simulink model "Attitude_Control"  (R2021b)
settings: Solver=VariableStepAuto  StartTime=0.0  StopTime=Inf  FixedStep=0.001  RelTol=1e-3
values from neighbouring files (symbols this model uses):
  pitch_c = param(39)    [get_full_state.m]
  roll_c_1 = param(40)    [get_full_state.m]
  roll_c_2 = param(41)    [get_full_state.m]
undefined symbols (not defined in the file or in its folder): k_pitch, k_roll
libraries: vrlib x6, simulink_extras x3, matrix_library x3
settings Model: Creator=austm  LastModifiedBy=austm
settings SolverCC: ZeroCrossAlgorithm=Adaptive  AlgebraicLoopSolver=TrustRegion  AutoInsertRateTranBlk=on  InsertRTBMode=Never (minimum delay)  DecoupledContinuousIntegration=on  MinimalZcImpactIntegration=on
settings DataIOCC: ExternalInput=inputs0  InitialState=states  SaveFormat=Array  SaveOutput=off  SaveTime=off  ReturnWorkspaceOutputsName=tpc05cf441_1fa6_4e1e_817c_7c8b4b7bc3e9
settings OptimizationCC: EnhancedBackFolding=on  StrengthReduction=on  InitFltsAndDblsToZero=on  DifferentSizesBufferReuse=on
settings DebuggingCC: WriteAfterWriteMsg=DisableAll  AlgebraicLoopMsg=none  IgnoredZcDiagnostic=none  FcnCallInpInsideContextMsg=warning  UnconnectedInputMsg=none  UnconnectedOutputMsg=none  UnconnectedLineMsg=none  UniqueDataStoreMsg=error  RootOutportRequireBusObject=none  StateNameClashWarn=warning  StrictBusMsg=ErrorOnBusTreatedAsVector  SFUnexpectedBacktrackingDiag=warning  SFNoUnconditionalDefaultTransitionDiag=warning  SFExecutionAtInitializationDiag=none  SFMachineParentedDataDiag=warning  ArithmeticOperatorsInVariantConditions=warning
settings ModelReferenceCC: PropagateSignalLabelsOutOfModel=off
settings SFSimCC: SimUseLocalCustomCode=off
settings RTWCC: RTWUseLocalCustomCode=off
settings CodeAppCC: StateflowObjectComments=on

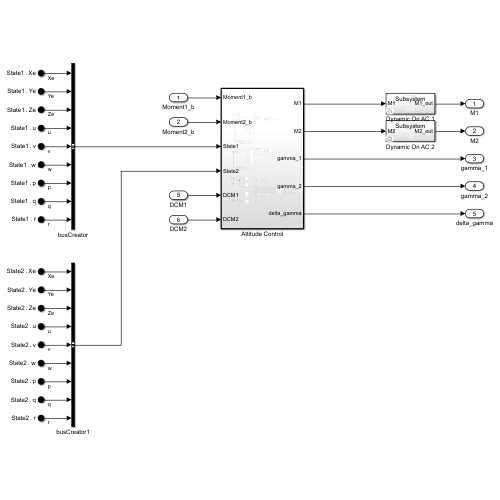
[thumbnail: Simulink's stored preview of the top-level diagram]
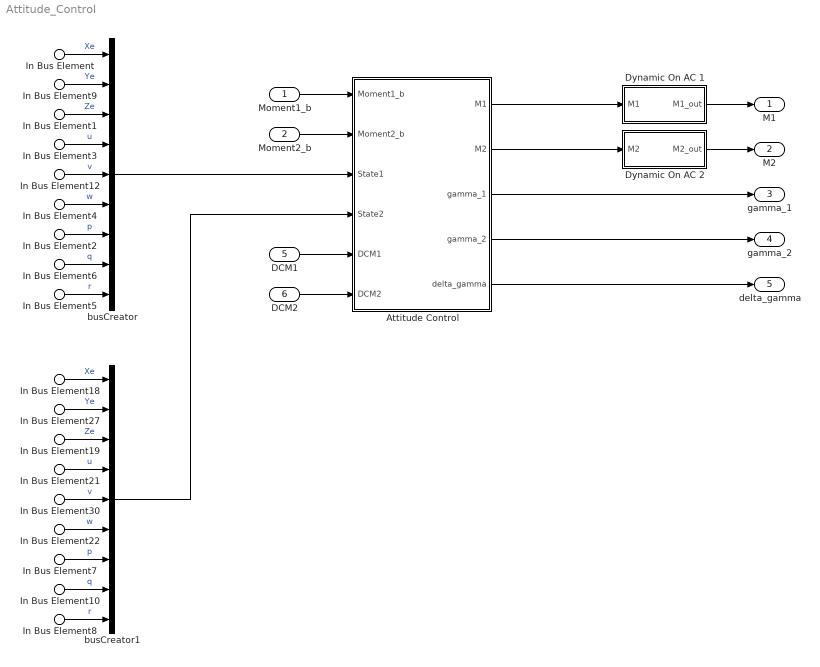
== system Attitude_Control ==
  Moment1_b : Inport  OutDataTypeStr=double  PortDimensions=3  SampleTime=0
  Moment2_b : Inport  Port=2  OutDataTypeStr=double  PortDimensions=3  SampleTime=0
  In Bus Element : Inport  Port=3  PortName=State1  Element=Xe
  In Bus Element1 : Inport  Port=3  PortName=State1  Element=Ze
  In Bus Element3 : Inport  Port=3  PortName=State1  Element=u
  In Bus Element4 : Inport  Port=3  PortName=State1  Element=w
  In Bus Element9 : Inport  Port=3  PortName=State1  Element=Ye
  In Bus Element12 : Inport  Port=3  PortName=State1  Element=v
  In Bus Element2 : Inport  Port=3  PortName=State1  Element=p
  In Bus Element6 : Inport  Port=3  PortName=State1  Element=q
  In Bus Element5 : Inport  Port=3  PortName=State1  Element=r
  In Bus Element18 : Inport  Port=4  PortName=State2  Element=Xe
  In Bus Element19 : Inport  Port=4  PortName=State2  Element=Ze
  In Bus Element21 : Inport  Port=4  PortName=State2  Element=u
  In Bus Element22 : Inport  Port=4  PortName=State2  Element=w
  In Bus Element27 : Inport  Port=4  PortName=State2  Element=Ye
  In Bus Element30 : Inport  Port=4  PortName=State2  Element=v
  In Bus Element7 : Inport  Port=4  PortName=State2  Element=p
  In Bus Element10 : Inport  Port=4  PortName=State2  Element=q
  In Bus Element8 : Inport  Port=4  PortName=State2  Element=r
  DCM1 : Inport  Port=5  OutDataTypeStr=double  PortDimensions=[3 3]  SampleTime=0
  DCM2 : Inport  Port=6  OutDataTypeStr=double  PortDimensions=[3 3]  SampleTime=0
  Attitude Control : Subsystem  TreatAsAtomicUnit=on
  Dynamic On AC 1 : Subsystem  Variant=on
  Dynamic On AC 2 : Subsystem  Variant=on
  busCreator : BusCreator  Inputs=9
  busCreator1 : BusCreator  Inputs=9
  M1 : Outport  OutDataTypeStr=double  PortDimensions=3  SampleTime=0
  M2 : Outport  Port=2  OutDataTypeStr=double  PortDimensions=3  SampleTime=0
  gamma_1 : Outport  Port=3  OutDataTypeStr=double  PortDimensions=3  SampleTime=0
  gamma_2 : Outport  Port=4  OutDataTypeStr=double  PortDimensions=3  SampleTime=0
  delta_gamma : Outport  Port=5  OutDataTypeStr=double  PortDimensions=3  SampleTime=0
  wires:
  DCM2/1 -> Attitude Control/6(DCM2)
  Moment1_b/1 -> Attitude Control/1(Moment1_b)
  Attitude Control/2(M2) -> Dynamic On AC 2/1(M2)
  DCM1/1 -> Attitude Control/5(DCM1)
  Attitude Control/1(M1) -> Dynamic On AC 1/1(M1)
  In Bus Element30/1 -> busCreator1/5  "v"
  In Bus Element27/1 -> busCreator1/2  "Ye"
  In Bus Element22/1 -> busCreator1/6  "w"
  In Bus Element21/1 -> busCreator1/4  "u"
  In Bus Element18/1 -> busCreator1/1  "Xe"
  In Bus Element19/1 -> busCreator1/3  "Ze"
  busCreator1/1 -> Attitude Control/4(State2)
  In Bus Element12/1 -> busCreator/5  "v"
  In Bus Element9/1 -> busCreator/2  "Ye"
  In Bus Element4/1 -> busCreator/6  "w"
  In Bus Element3/1 -> busCreator/4  "u"
  In Bus Element1/1 -> busCreator/3  "Ze"
  In Bus Element/1 -> busCreator/1  "Xe"
  busCreator/1 -> Attitude Control/3(State1)
  Moment2_b/1 -> Attitude Control/2(Moment2_b)
  Dynamic On AC 1/1(M1_out) -> M1/1
  Dynamic On AC 2/1(M2_out) -> M2/1
  In Bus Element2/1 -> busCreator/7  "p"
  In Bus Element6/1 -> busCreator/8  "q"
  In Bus Element5/1 -> busCreator/9  "r"
  In Bus Element7/1 -> busCreator1/7  "p"
  In Bus Element10/1 -> busCreator1/8  "q"
  In Bus Element8/1 -> busCreator1/9  "r"
  Attitude Control/3(gamma_1) -> gamma_1/1
  Attitude Control/4(gamma_2) -> gamma_2/1
  Attitude Control/5(delta_gamma) -> delta_gamma/1

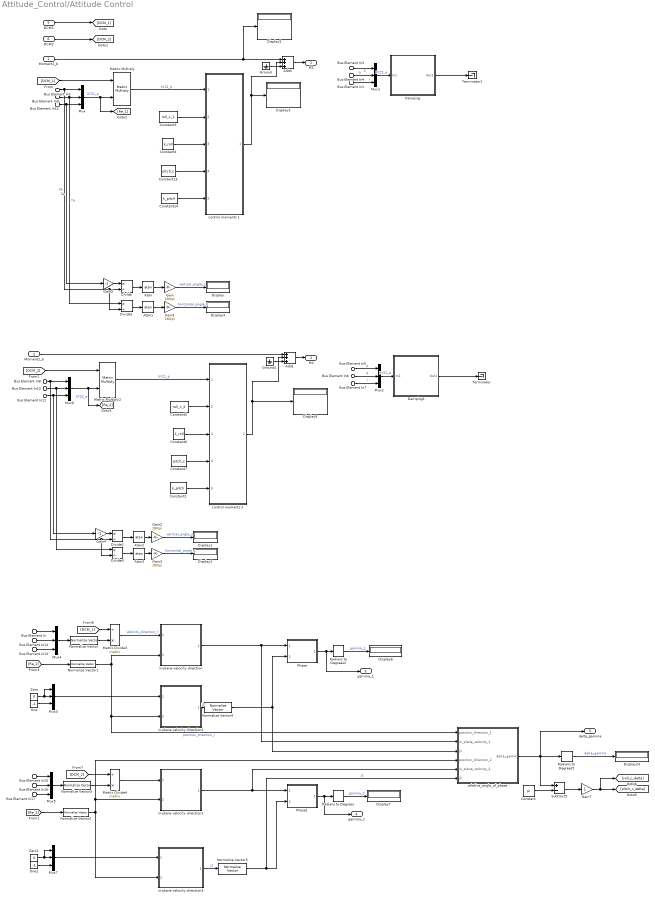
== system Attitude_Control/Attitude Control ==
  Moment1_b : Inport
  Moment2_b : Inport  Port=2
  Bus Element In12 : Inport  Port=3  PortName=State1  Element=Ze
  Bus Element In2 : Inport  Port=3  PortName=State1  Element=Xe
  Bus Element In9 : Inport  Port=3  PortName=State1  Element=Ye
  Bus Element In : Inport  Port=3  PortName=State1  Element=u
  Bus Element In13 : Inport  Port=3  PortName=State1  Element=w
  Bus Element In14 : Inport  Port=3  PortName=State1  Element=v
  Bus Element In3 : Inport  Port=3  PortName=State1  Element=p
  Bus Element In4 : Inport  Port=3  PortName=State1  Element=q
  Bus Element In1 : Inport  Port=3  PortName=State1  Element=r
  Bus Element In8 : Inport  Port=4  PortName=State2  Element=Xe
  Bus Element In10 : Inport  Port=4  PortName=State2  Element=Ye
  Bus Element In11 : Inport  Port=4  PortName=State2  Element=Ze
  Bus Element In15 : Inport  Port=4  PortName=State2  Element=u
  Bus Element In16 : Inport  Port=4  PortName=State2  Element=v
  Bus Element In17 : Inport  Port=4  PortName=State2  Element=w
  Bus Element In5 : Inport  Port=4  PortName=State2  Element=p
  Bus Element In6 : Inport  Port=4  PortName=State2  Element=q
  Bus Element In7 : Inport  Port=4  PortName=State2  Element=r
  DCM1 : Inport  Port=5
  DCM2 : Inport  Port=6
  Add1 : Sum  Inputs=+++
  Add3 : Sum  Inputs=+++
  Atan{,1..3} (4 alike) : Trigonometry  Operator=atan
  Constant : Constant  Value=pi
  Constant13 : Constant  Value=pitch_c
  Constant14 : Constant  Value=k_pitch
  Constant2 : Constant  Value=k_pitch
  Constant3 : Constant  Value=roll_c_1
  Constant4 : Constant  Value=k_roll
  Constant5 : Constant  Value=roll_c_2
  Constant6 : Constant  Value=k_roll
  Constant7 : Constant  Value=pitch_c
  Damping : Subsystem
  Damping1 : Subsystem
  Display{,1..8,24} (10 alike) : Display
  Divide{,1..3} (4 alike) : Product  Inputs=*/
  Gain{,1..3} (4 alike) : Gain  Gain=180/pi
  Gain4 : Gain  Gain=-1
  Gain5 : Gain  Gain=-1
  Gain7 : Gain
  Ground : Ground
  Ground1 : Ground
  Matrix Divide3 : Product  Inputs=/*  Multiplication=Matrix(*)
  Matrix Divide4 : Product  Inputs=/*  Multiplication=Matrix(*)
  Matrix Multiply : Product  Multiplication=Matrix(*)
  Matrix Multiply2 : Product  Multiplication=Matrix(*)
  Mux{,1..7} (8 alike) : Mux  Inputs=3
  Normalize Vector{,1..5} (6 alike) : vrlib/Utilities/Normalize Vector  maxzero=0
  One : Constant  Value=-1  OutDataTypeStr=Inherit: Inherit via back propagation
  One1 : Constant  Value=-1  OutDataTypeStr=Inherit: Inherit via back propagation
  Phase : Subsystem  ReferencedSubsystem=Phase
  Phase1 : Subsystem  ReferencedSubsystem=Phase
  Radians to Degrees : simulink_extras/Transformations/Radians to Degrees
  Radians to Degrees2 : simulink_extras/Transformations/Radians to Degrees
  Radians to Degrees5 : simulink_extras/Transformations/Radians to Degrees
  Subtract5 : Sum  Inputs=+-
  Terminator : Terminator
  Terminator1 : Terminator
  Zero : Constant  Value=0  OutDataTypeStr=Inherit: Inherit via back propagation
  Zero1 : Constant  Value=0  OutDataTypeStr=Inherit: Inherit via back propagation
  control moments 1 : Subsystem  ReferencedSubsystem=control_moments
  control moments 2 : Subsystem  ReferencedSubsystem=control_moments
  in-plane velocity direction{,1..3} (4 alike) : Subsystem  ReferencedSubsystem=in_plane_velocity_direction
  relative_angle_of_phase : Subsystem
  M1 : Outport
  M2 : Outport  Port=2
  gamma_1 : Outport  Port=3
  gamma_2 : Outport  Port=4
  delta_gamma : Outport  Port=5
  wires:
  relative_angle_of_phase/1(delta_gamma) -> delta_gamma/1, Subtract5/1, Radians to Degrees5/1
  Phase/1 -> gamma_1/1, Radians to Degrees2/1
  Mux7/1 -> in-plane velocity direction3/1
  Matrix Divide4/1 -> in-plane velocity direction1/1
  Mux3/1 -> in-plane velocity direction2/1
  in-plane velocity direction2/1 -> Normalize Vector4/1  "j1"
  Matrix Divide3/1 -> in-plane velocity direction/1  "velocity_direction_I"
  in-plane velocity direction/1 -> relative_angle_of_phase/2(in_plane_velocity_1), Phase/1
  Gain7/1 -> [pitch_c_delta], [roll_c_delta]
  Subtract5/1 -> Gain7/1
  Constant7/1 -> control moments 2/4
  Constant/1 -> Subtract5/2
  Radians to Degrees5/1 -> Display24/1  "delta_gamma"
  Normalize Vector1/1 -> in-plane velocity direction/2, in-plane velocity direction2/2, relative_angle_of_phase/1(position_direction_1)  "position_direction_I"
  Phase1/1 -> gamma_2/1, Radians to Degrees/1
  in-plane velocity direction1/1 -> relative_angle_of_phase/5(in_plane_velocity_2), Phase1/1
  Radians to Degrees/1 -> Display7/1  "gamma_2"
  Radians to Degrees2/1 -> Display6/1  "gamma_1"
  Normalize Vector5/1 -> Phase1/2, relative_angle_of_phase/6(j2)  "j2"
  Normalize Vector2/1 -> relative_angle_of_phase/4(position_direction_2), in-plane velocity direction1/2, in-plane velocity direction3/2
  One1/1 -> Mux7/3
  Zero1/1 -> Mux7/2, Mux7/1
  Zero/1 -> Mux3/2, Mux3/1
  One/1 -> Mux3/3
  Normalize Vector3/1 -> Matrix Divide4/2
  [Re_2] -> Normalize Vector2/1
  [Re_1] -> Normalize Vector1/1
  Normalize Vector/1 -> Matrix Divide3/2
  [DCM_1] -> Matrix Divide3/1
  Bus Element In14/1 -> Mux4/2
  [DCM_2] -> Matrix Divide4/1
  Mux5/1 -> Normalize Vector3/1
  Bus Element In17/1 -> Mux5/3
  Mux4/1 -> Normalize Vector/1
  Bus Element In/1 -> Mux4/1
  Bus Element In15/1 -> Mux5/1
  Bus Element In16/1 -> Mux5/2
  Bus Element In13/1 -> Mux4/3
  Atan/1 -> Gain/1
  Gain5/1 -> Divide/1
  Gain4/1 -> Divide2/1
  Gain2/1 -> Display1/1  "vertical_angle_2"
  Atan2/1 -> Gain2/1
  Atan3/1 -> Gain3/1
  Gain3/1 -> Display2/1  "horizontal_angle_2"
  Gain1/1 -> Display4/1  "horizontal_angle_1"
  Atan1/1 -> Gain1/1
  Gain/1 -> Display/1  "vertical_angle_1"
  Divide3/1 -> Atan3/1
  Divide2/1 -> Atan2/1
  Divide1/1 -> Atan1/1
  Divide/1 -> Atan/1
  Constant2/1 -> control moments 2/5
  Constant6/1 -> control moments 2/3
  Constant5/1 -> control moments 2/2
  Constant14/1 -> control moments 1/5
  Constant13/1 -> control moments 1/4
  Constant4/1 -> control moments 1/3
  Constant3/1 -> control moments 1/2
  control moments 2/1 -> Add1/2, Display8/1
  Matrix Multiply2/1 -> control moments 2/1  "XYZ1_b"
  Add3/1 -> M1/1
  control moments 1/1 -> Display3/1, Add3/2
  Matrix Multiply/1 -> control moments 1/1  "XYZ1_b"
  [DCM_2] -> Matrix Multiply2/1
  Bus Element In11/1 -> Mux6/3, Gain4/1
  Bus Element In10/1 -> Mux6/2, Divide3/1
  Bus Element In8/1 -> Mux6/1, Divide3/2, Divide2/2
  Add1/1 -> M2/1
  Mux6/1 -> Matrix Multiply2/2, [Re_2]  "XYZ2_e"
  Moment1_b/1 -> Add3/1, Display5/1
  DCM2/1 -> [DCM_2]
  DCM1/1 -> [DCM_1]
  Bus Element In2/1 -> Mux/1, Divide/2, Divide1/2  "Xe"
  Bus Element In12/1 -> Mux/3, Gain5/1  "Ze"
  Bus Element In9/1 -> Mux/2, Divide1/1  "Ye"
  Mux/1 -> Matrix Multiply/2, [Re_1]  "XYZ1_e"
  [DCM_1] -> Matrix Multiply/1
  Moment2_b/1 -> Add1/1
  Normalize Vector4/1 -> Phase/2, relative_angle_of_phase/3(j1)
  in-plane velocity direction3/1 -> Normalize Vector5/1  "j2"
  Bus Element In3/1 -> Mux1/1  "p"
  Bus Element In4/1 -> Mux1/2  "q"
  Bus Element In1/1 -> Mux1/3  "r"
  Mux1/1 -> Damping/1(In1)  "XYZ1_e"
  Damping/1(Out1) -> Terminator1/1
  Mux2/1 -> Damping1/1(In1)  "XYZ1_e"
  Bus Element In6/1 -> Mux2/2  "q"
  Bus Element In7/1 -> Mux2/3  "r"
  Bus Element In5/1 -> Mux2/1  "p"
  Damping1/1(Out1) -> Terminator/1
  Ground/1 -> Add3/3
  Ground1/1 -> Add1/3

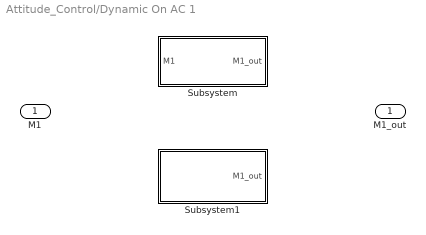
== system Attitude_Control/Dynamic On AC 1 ==
  M1 : Inport
  Subsystem : Subsystem  VariantControl=ac1_moments > 0
  Subsystem1 : Subsystem  VariantControl="ac1_moments ==  0"
  M1_out : Outport

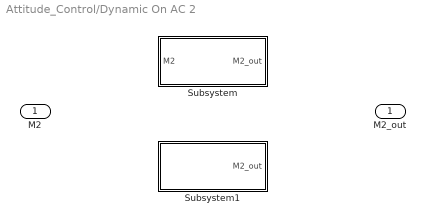
== system Attitude_Control/Dynamic On AC 2 ==
  M2 : Inport
  Subsystem : Subsystem  VariantControl=ac2_moments > 0
  Subsystem1 : Subsystem  VariantControl=ac2_moments == 0
  M2_out : Outport

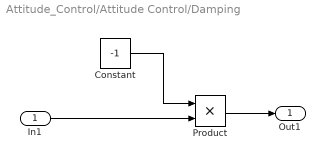
== system Attitude_Control/Attitude Control/Damping ==
  In1 : Inport
  Constant : Constant  Value=-1
  Product : Product
  Out1 : Outport
  wires:
  In1/1 -> Product/2
  Product/1 -> Out1/1
  Constant/1 -> Product/1

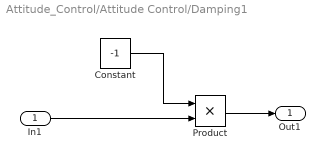
== system Attitude_Control/Attitude Control/Damping1 ==
  In1 : Inport
  Constant : Constant  Value=-1
  Product : Product
  Out1 : Outport
  wires:
  In1/1 -> Product/2
  Product/1 -> Out1/1
  Constant/1 -> Product/1

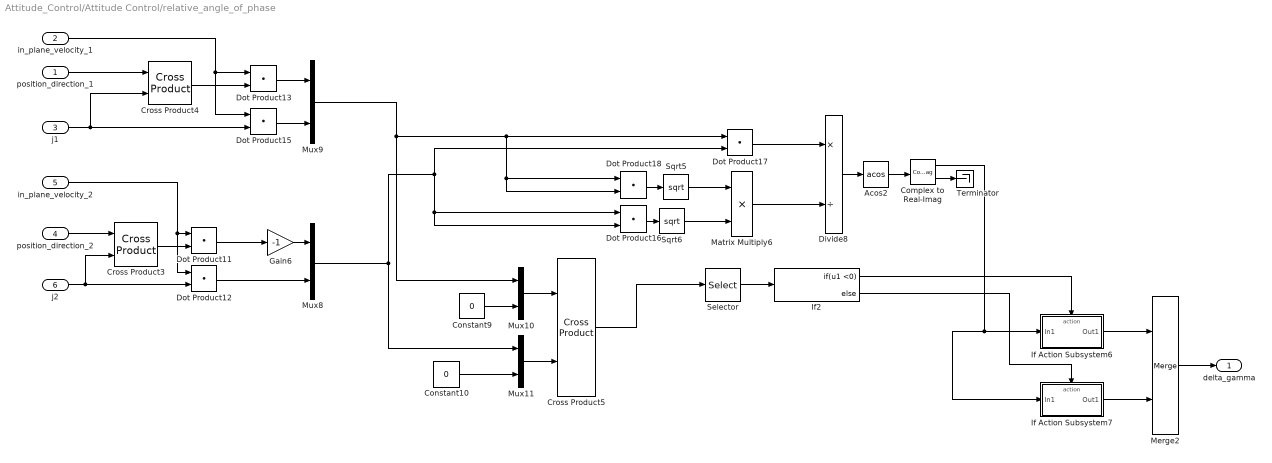
== system Attitude_Control/Attitude Control/relative_angle_of_phase ==
  position_direction_1 : Inport
  in_plane_velocity_1 : Inport  Port=2
  j1 : Inport  Port=3
  position_direction_2 : Inport  Port=4
  in_plane_velocity_2 : Inport  Port=5
  j2 : Inport  Port=6
  Acos2 : Trigonometry  Operator=acos  OutputSignalType=complex
  Complex to Real-Imag : ComplexToRealImag
  Constant10 : Constant  Value=0
  Constant9 : Constant  Value=0
  Cross Product3 : matrix_library/Cross Product
      settings: SourceProductBaseCode=SL
  Cross Product4 : matrix_library/Cross Product
      settings: SourceProductBaseCode=SL
  Cross Product5 : matrix_library/Cross Product
      settings: SourceProductBaseCode=SL
  Divide8 : Product  Inputs=*/
  Dot Product{11..13,15..18} (7 alike) : DotProduct  InputSameDT=on  OutDataTypeStr=Inherit: Inherit via internal rule
  Gain6 : Gain  Gain=-1
  If Action Subsystem6 : Subsystem  TreatAsAtomicUnit=on
  If Action Subsystem7 : Subsystem  TreatAsAtomicUnit=on
  If2 : If  IfExpression=u1 <0
  Matrix Multiply6 : Product
  Merge2 : Merge
  Mux{8..11} (4 alike) : Mux  Inputs=2
  Selector : Selector  InputPortWidth=3  IndexOptions=Index vector (dialog)  Indices=3  OutputSizes=1
  Sqrt5 : Sqrt  SaturateOnIntegerOverflow=on
  Sqrt6 : Sqrt  SaturateOnIntegerOverflow=on
  Terminator : Terminator
  delta_gamma : Outport
  wires:
  Acos2/1 -> Complex to Real-Imag/1
  Complex to Real-Imag/2 -> Terminator/1
  j1/1 -> Dot Product15/2, Cross Product4/2
  If Action Subsystem7/1(Out1) -> Merge2/2
  Dot Product15/1 -> Mux9/2
  If Action Subsystem6/1(Out1) -> Merge2/1
  Mux10/1 -> Cross Product5/1
  Constant9/1 -> Mux10/2
  Dot Product17/1 -> Divide8/1
  Cross Product5/1 -> Selector/1
  j2/1 -> Dot Product12/2, Cross Product3/2
  Mux11/1 -> Cross Product5/2
  Dot Product16/1 -> Sqrt6/1
  Merge2/1 -> delta_gamma/1
  in_plane_velocity_1/1 -> Dot Product15/1, Dot Product13/1
  If2/1 -> If Action Subsystem6/Action
  Sqrt6/1 -> Matrix Multiply6/2
  position_direction_2/1 -> Cross Product3/1
  Sqrt5/1 -> Matrix Multiply6/1
  Complex to Real-Imag/1 -> If Action Subsystem6/1(In1), If Action Subsystem7/1(In1)
  position_direction_1/1 -> Cross Product4/1
  Matrix Multiply6/1 -> Divide8/2
  Cross Product4/1 -> Dot Product13/2
  Divide8/1 -> Acos2/1
  Gain6/1 -> Mux8/1
  Selector/1 -> If2/1
  Dot Product18/1 -> Sqrt5/1
  Cross Product3/1 -> Dot Product11/2
  Mux8/1 -> Mux11/1, Dot Product17/2, Dot Product16/1, Dot Product16/2
  Dot Product12/1 -> Mux8/2
  Constant10/1 -> Mux11/2
  Dot Product11/1 -> Gain6/1
  If2/2 -> If Action Subsystem7/Action
  in_plane_velocity_2/1 -> Dot Product11/1, Dot Product12/1
  Dot Product13/1 -> Mux9/1
  Mux9/1 -> Mux10/1, Dot Product17/1, Dot Product18/1, Dot Product18/2

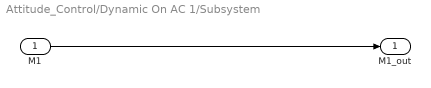
== system Attitude_Control/Dynamic On AC 1/Subsystem ==
  M1 : Inport
  M1_out : Outport
  wires:
  M1/1 -> M1_out/1

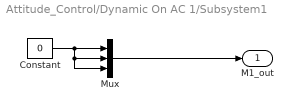
== system Attitude_Control/Dynamic On AC 1/Subsystem1 ==
  Constant : Constant  Value=0
  Mux : Mux  Inputs=3
  M1_out : Outport
  wires:
  Mux/1 -> M1_out/1
  Constant/1 -> Mux/3, Mux/2, Mux/1

== system Attitude_Control/Dynamic On AC 2/Subsystem ==
  M2 : Inport
  M2_out : Outport
  wires:
  M2/1 -> M2_out/1

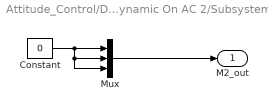
== system Attitude_Control/Dynamic On AC 2/Subsystem1 ==
  Constant : Constant  Value=0
  Mux : Mux  Inputs=3
  M2_out : Outport
  wires:
  Constant/1 -> Mux/3, Mux/2, Mux/1
  Mux/1 -> M2_out/1

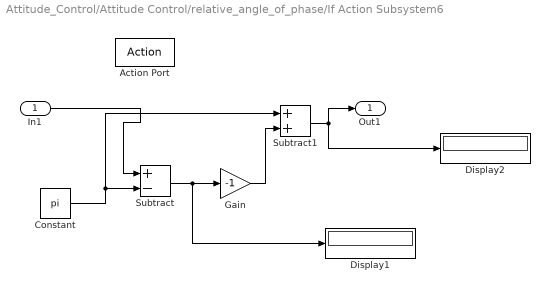
== system Attitude_Control/Attitude Control/relative_angle_of_phase/If Action Subsystem6 ==
  In1 : Inport
  Action Port : ActionPort  ActionPortLabel=if(u1 <0)
  Constant : Constant  Value=pi
  Display1 : Display
  Display2 : Display
  Gain : Gain  Gain=-1
  Subtract : Sum  Inputs=+-
  Subtract1 : Sum
  Out1 : Outport
  wires:
  Constant/1 -> Subtract/2, Subtract1/1
  Subtract1/1 -> Display2/1, Out1/1
  Gain/1 -> Subtract1/2
  Subtract/1 -> Gain/1, Display1/1
  In1/1 -> Subtract/1

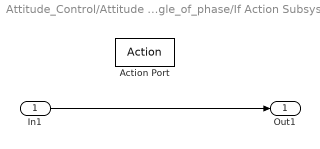
== system Attitude_Control/Attitude Control/relative_angle_of_phase/If Action Subsystem7 ==
  In1 : Inport
  Action Port : ActionPort  ActionPortLabel=else
  Out1 : Outport
  wires:
  In1/1 -> Out1/1
